simulink model "exsim5model"  (Simulink 7.2)
settings: Solver=ode45  StartTime=0.0  StopTime=tf  FixedStep=T  RelTol=1e-3
values from neighbouring files (symbols this model uses):
  a = 7/(4*T)    [controller.m]    (also in exsim2script.m = 2; exsim5script.m = 2)
  alpha = (kp*T^2)/(2*J)    (= 0.98)    [exsim2script.m]    (also in exsim5script.m)
  b = 2/(5*T)    [controller.m]    (also in exsim2script.m = 0.5; exsim5script.m = 0.5)
  J = 1    [exsim2script.m]    (also in exsim5script.m)
  kc = 5/(4*alpha)    [controller.m]    (also in exsim2script.m = 2; exsim5script.m = 2)
  kp = 1    [exsim2script.m]    (also in exsim5script.m)
  r1 = 0.75    [controller2.m]    (also in ctrld.m; exsim2script.m; exsim5script.m)
  s0 = 1.25/alpha    [controller2.m]    (also in ctrld.m; exsim2script.m = 1.27551020408; exsim5script.m = 1.27551020408)
  s1 = -0.75/alpha    [controller2.m]    (also in ctrld.m; exsim2script.m = -0.765306122449; exsim5script.m = -0.765306122449)
  T = 1.4/w0    (= 1.4)    [exsim2script.m]    (also in exsim5script.m)
  t0 = 1/(2*alpha)    [controller2.m]    (also in ctrld.m; exsim2script.m = 0.510204081633; exsim5script.m = 0.510204081633)
settings Model: Creator=hcf2k  LastModifiedBy=hcf2k  CovModelRefEnable=off
settings DataIOCC: SaveFormat=StructureWithTime
settings OptimizationCC: ExpressionDepthLimit=128
settings DebuggingCC: UnderspecifiedInitializationDetection=Simplified  MergeDetectMultiDrivingBlocksExec=error  SolverPrmCheckMsg=none  FcnCallInpInsideContextMsg=Enable All  StateNameClashWarn=none  StrictBusMsg=ErrorLevel1
settings HardwareCC: ProdIntDivRoundTo=Zero  ProdEndianess=LittleEndian  ProdHWDeviceType=Specified
settings CodeAppCC: CustomSymbolStrType=$N$R$M_T
settings GRTTargetCC: TargetFunctionLibrary=C89/C90 (ANSI)

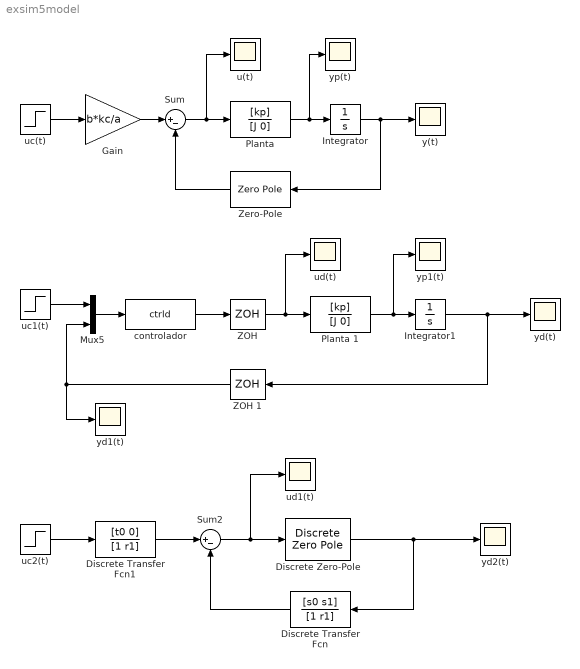
== system exsim5model ==
  Discrete Transfer Fcn : DiscreteTransferFcn  Orientation=left  Numerator=[s0 s1]  Denominator=[1 r1]
  Discrete Transfer Fcn1 : DiscreteTransferFcn  Numerator=[t0 0]  Denominator=[1 r1]
  Discrete Zero-Pole : DiscreteZeroPole  Zeros=[-1]  Poles=[1 1]  Gain=alpha  SampleTime=T
  Gain : Gain  Gain=b*kc/a
  Integrator : Integrator
  Integrator1 : Integrator
  Mux5 : Mux  Inputs=2
  Planta : TransferFcn  Numerator=[kp]  Denominator=[J 0]
  Planta 1 : TransferFcn  Numerator=[kp]  Denominator=[J 0]
  Sum : Sum  Inputs=|+-
  Sum2 : Sum  Inputs=|+-
  ZOH : ZeroOrderHold  SampleTime=T
  ZOH 1 : ZeroOrderHold  Orientation=left  SampleTime=T
  Zero-Pole : ZeroPole  Orientation=left  Zeros=[-b]  Poles=[-a]  Gain=[kc]
  controlador : MATLABFcn  MATLABFcn=ctrld  OutputDimensions=1
  u(t) : Scope
      settings: TimeRange=auto  MaxDataPoints=5000  SaveName=u  YMin=-0.63776  YMax=0.63776  SampleTime=-1  DataFormat=Array
  uc(t) : Step  Time=0  SampleTime=0
  uc1(t) : Step  Time=0  SampleTime=T
  uc2(t) : Step  Time=0  SampleTime=T
  ud(t) : Scope
      settings: TimeRange=auto  MaxDataPoints=5000  SaveName=ud  YMin=-0.63776  YMax=0.63776  SampleTime=-1  DataFormat=Array
  ud1(t) : Scope
      settings: TimeRange=auto  MaxDataPoints=5000  SaveName=ud1  YMin=-0.63776  YMax=0.63776  SampleTime=-1  DataFormat=Array
  y(t) : Scope
      settings: TimeRange=auto  MaxDataPoints=5000  SaveName=y  YMin=-0.1371  YMax=1.23391  SampleTime=-1  DataFormat=Array
  yd(t) : Scope
      settings: TimeRange=auto  MaxDataPoints=5000  SaveName=yd  YMin=-0.1371  YMax=1.23391  SampleTime=-1  DataFormat=Array
  yd1(t) : Scope
      settings: TimeRange=auto  MaxDataPoints=5000  SaveName=yd1  YMin=-0.125  YMax=1.125  SampleTime=-1  DataFormat=Array
  yd2(t) : Scope
      settings: TimeRange=auto  MaxDataPoints=5000  SaveName=yd2  YMin=-0.125  YMax=1.125  SampleTime=-1
  yp(t) : Scope
      settings: TimeRange=auto  MaxDataPoints=5000  SaveName=yp  YMin=-0.63776  YMax=0.63776  SampleTime=-1  DataFormat=Array
  yp1(t) : Scope
      settings: TimeRange=auto  MaxDataPoints=5000  SaveName=yp1  YMin=-0.63776  YMax=0.63776  SampleTime=-1  DataFormat=Array
  wires:
  Sum/1 -> u(t)/1, Planta/1
  Gain/1 -> Sum/1
  Zero-Pole/1 -> Sum/2
  uc(t)/1 -> Gain/1
  Integrator/1 -> y(t)/1, Zero-Pole/1
  Planta/1 -> yp(t)/1, Integrator/1
  controlador/1 -> ZOH/1
  ZOH/1 -> ud(t)/1, Planta 1/1
  Mux5/1 -> controlador/1
  ZOH 1/1 -> yd1(t)/1, Mux5/2
  uc1(t)/1 -> Mux5/1
  Planta 1/1 -> yp1(t)/1, Integrator1/1
  Integrator1/1 -> yd(t)/1, ZOH 1/1
  uc2(t)/1 -> Discrete Transfer Fcn1/1
  Discrete Transfer Fcn1/1 -> Sum2/1
  Sum2/1 -> Discrete Zero-Pole/1, ud1(t)/1
  Discrete Transfer Fcn/1 -> Sum2/2
  Discrete Zero-Pole/1 -> yd2(t)/1, Discrete Transfer Fcn/1
